simulink model "FTreal"  (Simulink 8.5)
settings: Solver=ode4  StartTime=0.0  StopTime=7  FixedStep=0.001  RelTol=1e-3
settings Model: Creator=guima  LastModifiedBy=guima
settings OptimizationCC: ExpressionDepthLimit=128  InitFltsAndDblsToZero=on
settings DebuggingCC: SaveWithParameterizedLinksMsg=none  SignalResolutionControl=TryResolveAllWithWarning  SolverPrmCheckMsg=warning  MultiTaskDSMMsg=warning  MultiTaskCondExecSysMsg=none  FcnCallInpInsideContextMsg=UseLocalSettings  StateNameClashWarn=none
settings GRTTargetCC: TargetFcnLib=ansi_tfl_tmw.mat

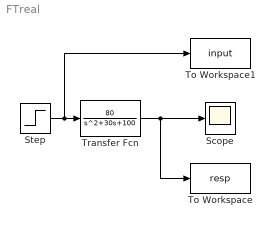
== system FTreal ==
  Scope : Scope
      settings: MaxDataPoints=7001
  Step : Step  Time=0  SampleTime=0
  To Workspace : ToWorkspace  VariableName=resp  SaveFormat=Structure With Time  SampleTime=-1
  To Workspace1 : ToWorkspace  VariableName=input  SaveFormat=Structure With Time  SampleTime=-1
  Transfer Fcn : TransferFcn  Numerator=[80]  Denominator=[1 30 100]
  wires:
  Step/1 -> Transfer Fcn/1, To Workspace1/1
  Transfer Fcn/1 -> Scope/1, To Workspace/1
